simulink model "untitled1"  (Simulink 7.5)
settings: Solver=ode45  StartTime=0.0  StopTime=10.0  RelTol=1e-3
libraries: simulink x4
settings Model: Creator=dell  LastModifiedBy=dell

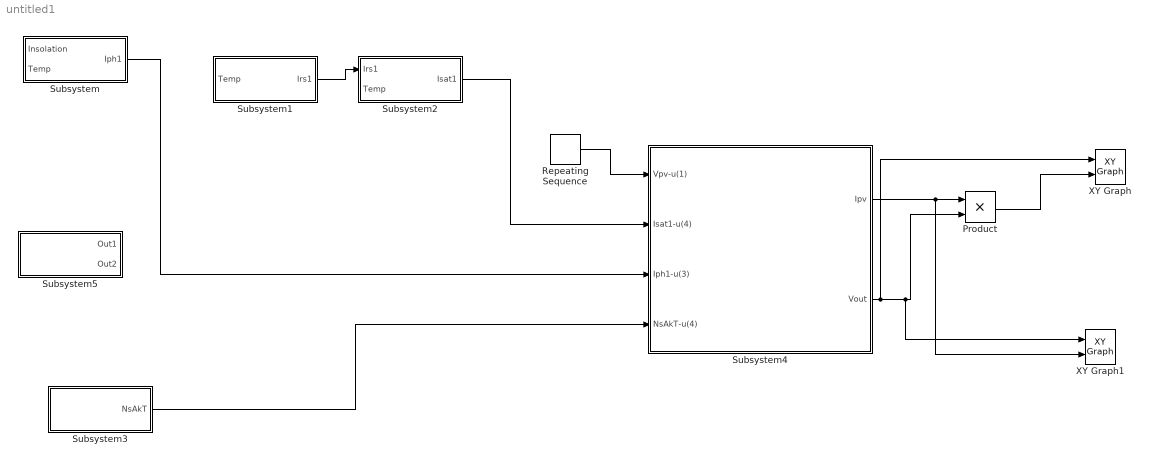
== system untitled1 ==
  Product : Product  OutDataType=fixdt(1, 16)  OutScaling=2^0  RndMeth=Zero
  Repeating Sequence : simulink/Sources/Repeating Sequence  SystemSampleTime=-1  rep_seq_t=[0 12]  rep_seq_y=[0 21.74]
  Subsystem : Subsystem
  Subsystem1 : Subsystem
  Subsystem2 : Subsystem
  Subsystem3 : Subsystem
  Subsystem4 : Subsystem
  Subsystem5 : Subsystem
  XY Graph : simulink/Sinks/XY Graph  SystemSampleTime=-1  xmin=0  xmax=25  ymin=0  ymax=40  st=-1
  XY Graph1 : simulink/Sinks/XY Graph  SystemSampleTime=-1  xmin=0  xmax=25  ymin=0  ymax=5  st=-1
  wires:
  Subsystem/1(Iph1) -> Subsystem4/3(Iph1-u(3))
  Subsystem1/1(Irs1) -> Subsystem2/1(Irs1)
  Subsystem3/1(NsAkT) -> Subsystem4/4(NsAkT-u(4))
  Subsystem2/1(Isat1) -> Subsystem4/2(Isat1-u(4))
  Repeating Sequence/1 -> Subsystem4/1(Vpv-u(1))
  Subsystem4/1(Ipv) -> Product/1, XY Graph1/2
  Subsystem4/2(Vout) -> Product/2, XY Graph1/1, XY Graph/1
  Product/1 -> XY Graph/2

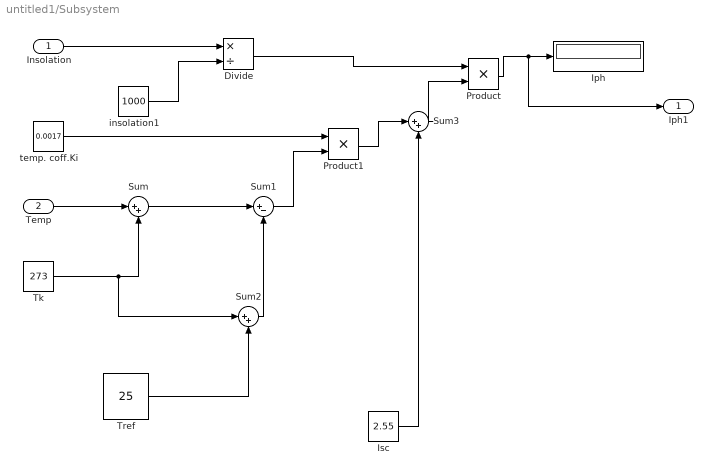
== system untitled1/Subsystem ==
  Insolation : Inport  OutDataType=fixdt(1, 16)  OutScaling=2^0
  Temp : Inport  Port=2  OutDataType=fixdt(1, 16)  OutScaling=2^0
  Divide : Product  Inputs=*/  OutDataType=fixdt(1, 16)  OutScaling=2^-10
  Iph : Display
  Isc : Constant  Value=2.55  OutDataType=fixdt(1, 16)  OutScaling=2^0
  Product : Product  OutDataType=fixdt(1, 16)  OutScaling=2^0  RndMeth=Zero
  Product1 : Product  OutDataType=fixdt(1, 16)  OutScaling=2^0  RndMeth=Zero
  Sum : Sum  Inputs=|++  OutDataType=fixdt(1, 16)  OutScaling=2^0
  Sum1 : Sum  Inputs=|+-  OutDataType=fixdt(1, 16)  OutScaling=2^0
  Sum2 : Sum  Inputs=|++  OutDataType=fixdt(1, 16)  OutScaling=2^0
  Sum3 : Sum  Inputs=|++  OutDataType=fixdt(1, 16)  OutScaling=2^0
  Tk : Constant  Value=273  OutDataType=fixdt(1, 16)  OutScaling=2^0
  Tref : Constant  Value=25  OutDataType=fixdt(1, 16)  OutScaling=2^0
  insolation1 : Constant  Value=1000  OutDataType=fixdt(1, 16)  OutScaling=2^0
  temp. coff.Ki : Constant  Value=0.0017  OutDataType=fixdt(1, 16)  OutScaling=2^0
  Iph1 : Outport  OutDataType=fixdt(1, 16)  OutScaling=2^0
  wires:
  Product/1 -> Iph/1, Iph1/1
  temp. coff.Ki/1 -> Product1/1
  Temp/1 -> Sum/1
  Tk/1 -> Sum/2, Sum2/1
  Sum/1 -> Sum1/1
  Tref/1 -> Sum2/2
  Sum2/1 -> Sum1/2
  Sum1/1 -> Product1/2
  Product1/1 -> Sum3/1
  Isc/1 -> Sum3/2
  Sum3/1 -> Product/2
  Insolation/1 -> Divide/1
  Divide/1 -> Product/1
  insolation1/1 -> Divide/2

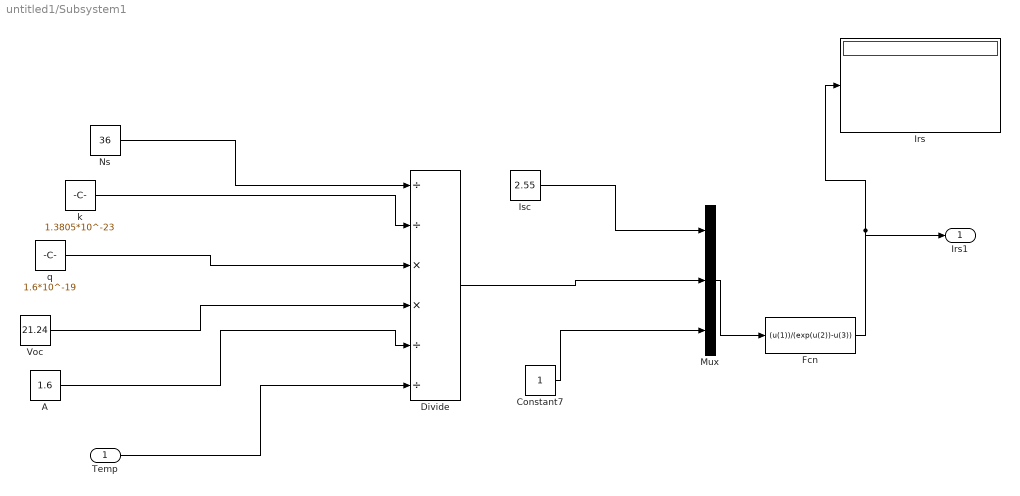
== system untitled1/Subsystem1 ==
  Temp : Inport  OutDataType=fixdt(1, 16)  OutScaling=2^0
  A : Constant  Value=1.6  OutDataType=fixdt(1, 16)  OutScaling=2^0
  Constant7 : Constant  OutDataType=fixdt(1, 16)  OutScaling=2^0
  Divide : Product  Inputs=//**//  OutDataType=fixdt(1, 16)  OutScaling=2^-10
  Fcn : Fcn  Expr=(u(1))/(exp(u(2))-u(3))
  Irs : Display
      settings: Format=short_e
  Isc : Constant  Value=2.55  OutDataType=fixdt(1, 16)  OutScaling=2^0
  Mux : Mux  Inputs=3
  Ns : Constant  Value=36  OutDataType=fixdt(1, 16)  OutScaling=2^0
  Voc : Constant  Value=21.24  OutDataType=fixdt(1, 16)  OutScaling=2^0
  k : Constant  Value=1.3805*10^-23  OutDataType=fixdt(1, 16)  OutScaling=2^0
  q : Constant  Value=1.6*10^-19  OutDataType=fixdt(1, 16)  OutScaling=2^0
  Irs1 : Outport  OutDataType=fixdt(1, 16)  OutScaling=2^0
  wires:
  Ns/1 -> Divide/1
  k/1 -> Divide/2
  q/1 -> Divide/3
  Voc/1 -> Divide/4
  A/1 -> Divide/5
  Temp/1 -> Divide/6
  Isc/1 -> Mux/1
  Divide/1 -> Mux/2
  Mux/1 -> Fcn/1
  Fcn/1 -> Irs/1, Irs1/1
  Constant7/1 -> Mux/3

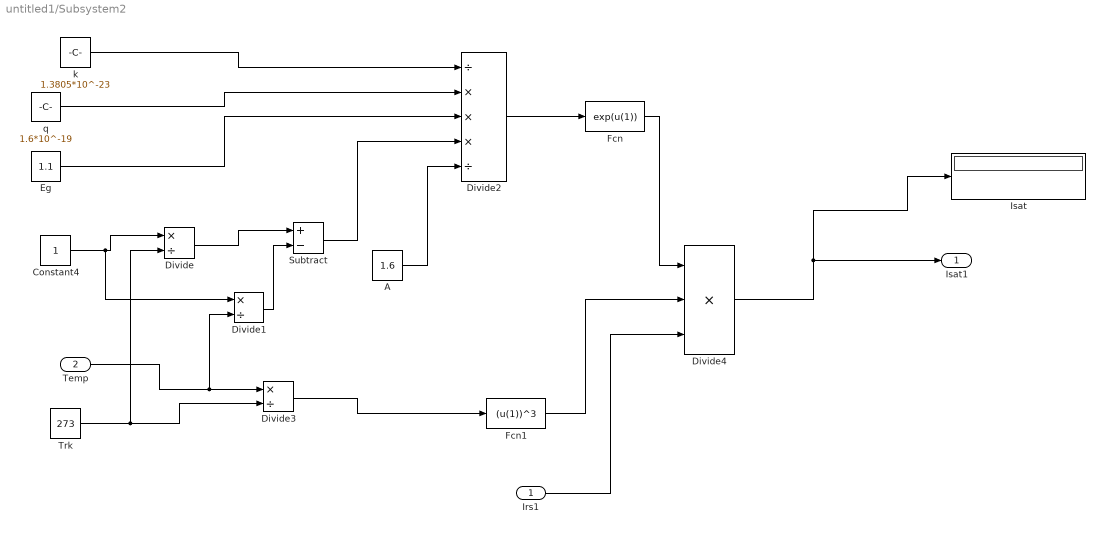
== system untitled1/Subsystem2 ==
  Irs1 : Inport  OutDataType=fixdt(1, 16)  OutScaling=2^0
  Temp : Inport  Port=2  OutDataType=fixdt(1, 16)  OutScaling=2^0
  A : Constant  Value=1.6  OutDataType=fixdt(1, 16)  OutScaling=2^0
  Constant4 : Constant  OutDataType=fixdt(1, 16)  OutScaling=2^0
  Divide : Product  Inputs=*/  OutDataType=fixdt(1, 16)  OutScaling=2^-10
  Divide1 : Product  Inputs=*/  OutDataType=fixdt(1, 16)  OutScaling=2^-10
  Divide2 : Product  Inputs=/***/  OutDataType=fixdt(1, 16)  OutScaling=2^-10
  Divide3 : Product  Inputs=*/  OutDataType=fixdt(1, 16)  OutScaling=2^-10
  Divide4 : Product  Inputs=***  OutDataType=fixdt(1, 16)  OutScaling=2^-10
  Eg : Constant  Value=1.1  OutDataType=fixdt(1, 16)  OutScaling=2^0
  Fcn : Fcn  Expr=exp(u(1))
  Fcn1 : Fcn  Expr=(u(1))^3
  Isat : Display
  Subtract : Sum  Inputs=+-  OutDataType=fixdt(1, 16)  OutScaling=2^-10
  Trk : Constant  Value=273  OutDataType=fixdt(1, 16)  OutScaling=2^0
  k : Constant  Value=1.3805*10^-23  OutDataType=fixdt(1, 16)  OutScaling=2^0
  q : Constant  Value=1.6*10^-19  OutDataType=fixdt(1, 16)  OutScaling=2^0
  Isat1 : Outport  OutDataType=fixdt(1, 16)  OutScaling=2^0
  wires:
  k/1 -> Divide2/1
  q/1 -> Divide2/2
  Eg/1 -> Divide2/3
  Constant4/1 -> Divide/1, Divide1/1
  Temp/1 -> Divide3/1, Divide1/2
  Trk/1 -> Divide3/2, Divide/2
  Divide/1 -> Subtract/1
  Divide1/1 -> Subtract/2
  Subtract/1 -> Divide2/4
  A/1 -> Divide2/5
  Divide2/1 -> Fcn/1
  Divide4/1 -> Isat/1, Isat1/1
  Fcn/1 -> Divide4/1
  Divide3/1 -> Fcn1/1
  Fcn1/1 -> Divide4/2
  Irs1/1 -> Divide4/3

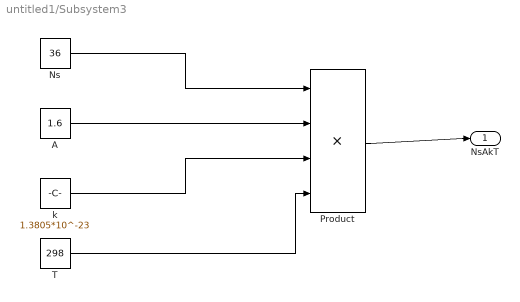
== system untitled1/Subsystem3 ==
  A : Constant  Value=1.6  OutDataType=fixdt(1, 16)  OutScaling=2^0
  Ns : Constant  Value=36  OutDataType=fixdt(1, 16)  OutScaling=2^0
  Product : Product  Inputs=4  OutDataType=fixdt(1, 16)  OutScaling=2^0  RndMeth=Zero
  T : Constant  Value=298  OutDataType=fixdt(1, 16)  OutScaling=2^0
  k : Constant  Value=1.3805*10^-23  OutDataType=fixdt(1, 16)  OutScaling=2^0
  NsAkT : Outport  OutDataType=fixdt(1, 16)  OutScaling=2^0
  wires:
  Ns/1 -> Product/1
  A/1 -> Product/2
  k/1 -> Product/3
  T/1 -> Product/4
  Product/1 -> NsAkT/1

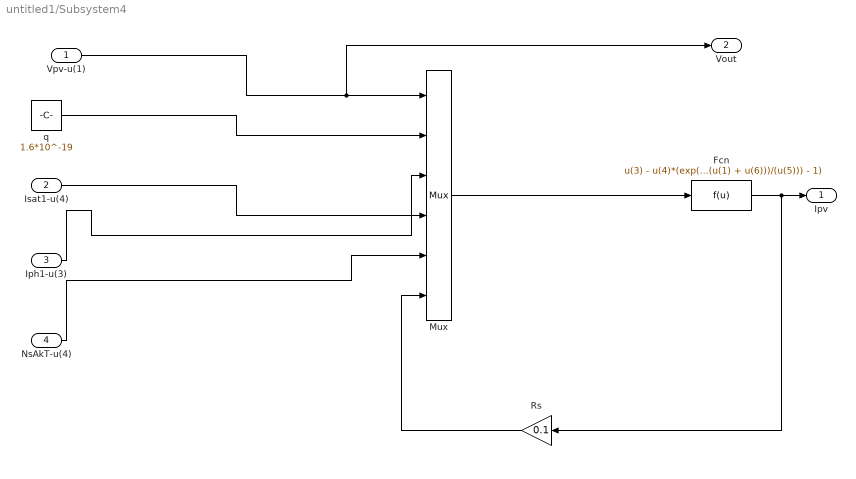
== system untitled1/Subsystem4 ==
  Vpv-u(1) : Inport  OutDataType=fixdt(1, 16)  OutScaling=2^0
  Isat1-u(4) : Inport  Port=2  OutDataType=fixdt(1, 16)  OutScaling=2^0
  Iph1-u(3) : Inport  Port=3  OutDataType=fixdt(1, 16)  OutScaling=2^0
  NsAkT-u(4) : Inport  Port=4  OutDataType=fixdt(1, 16)  OutScaling=2^0
  Fcn : Fcn  Expr=u(3) - u(4)*(exp((u(2)*(u(1) + u(6)))/(u(5))) - 1)
  Mux : Mux  Inputs=6
  Rs : Gain  Gain=0.1  ParameterDataType=fixdt(1, 16)  ParameterScaling=2^0  OutDataType=fixdt(1, 16)  OutScaling=2^0
  q : Constant  Value=1.6*10^-19  OutDataType=fixdt(1, 16)  OutScaling=2^0
  Ipv : Outport  OutDataType=fixdt(1, 16)  OutScaling=2^0
  Vout : Outport  Port=2  OutDataType=fixdt(1, 16)  OutScaling=2^0
  wires:
  Vpv-u(1)/1 -> Mux/1, Vout/1
  q/1 -> Mux/2
  NsAkT-u(4)/1 -> Mux/5
  Mux/1 -> Fcn/1
  Fcn/1 -> Ipv/1, Rs/1
  Isat1-u(4)/1 -> Mux/4
  Iph1-u(3)/1 -> Mux/3
  Rs/1 -> Mux/6

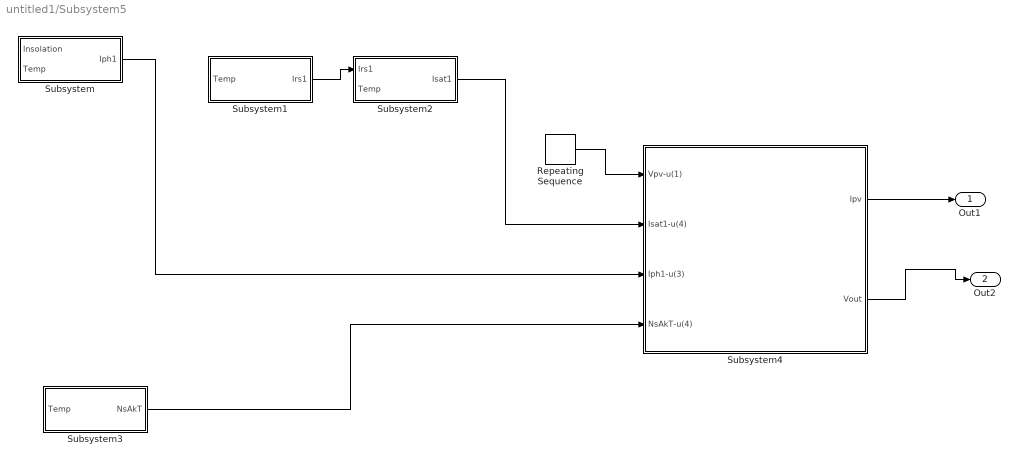
== system untitled1/Subsystem5 ==
  Repeating Sequence : simulink/Sources/Repeating Sequence  SystemSampleTime=-1  rep_seq_t=[0 12]  rep_seq_y=[0 21.74]
  Subsystem : Subsystem
  Subsystem1 : Subsystem
  Subsystem2 : Subsystem
  Subsystem3 : Subsystem
  Subsystem4 : Subsystem
  Out1 : Outport  OutDataType=fixdt(1, 16)  OutScaling=2^0
  Out2 : Outport  Port=2  OutDataType=fixdt(1, 16)  OutScaling=2^0
  wires:
  Subsystem/1(Iph1) -> Subsystem4/3(Iph1-u(3))
  Subsystem1/1(Irs1) -> Subsystem2/1(Irs1)
  Subsystem3/1(NsAkT) -> Subsystem4/4(NsAkT-u(4))
  Subsystem2/1(Isat1) -> Subsystem4/2(Isat1-u(4))
  Repeating Sequence/1 -> Subsystem4/1(Vpv-u(1))
  Subsystem4/1(Ipv) -> Out1/1
  Subsystem4/2(Vout) -> Out2/1

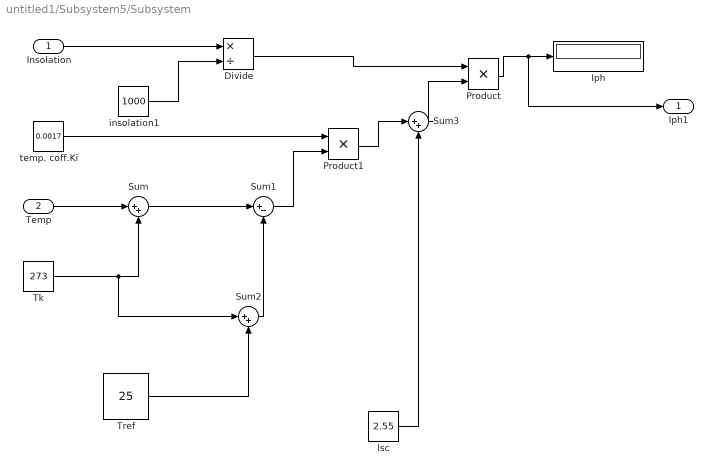
== system untitled1/Subsystem5/Subsystem ==
  Insolation : Inport  OutDataType=fixdt(1, 16)  OutScaling=2^0
  Temp : Inport  Port=2  OutDataType=fixdt(1, 16)  OutScaling=2^0
  Divide : Product  Inputs=*/  OutDataType=fixdt(1, 16)  OutScaling=2^-10
  Iph : Display
  Isc : Constant  Value=2.55  OutDataType=fixdt(1, 16)  OutScaling=2^0
  Product : Product  OutDataType=fixdt(1, 16)  OutScaling=2^0  RndMeth=Zero
  Product1 : Product  OutDataType=fixdt(1, 16)  OutScaling=2^0  RndMeth=Zero
  Sum : Sum  Inputs=|++  OutDataType=fixdt(1, 16)  OutScaling=2^0
  Sum1 : Sum  Inputs=|+-  OutDataType=fixdt(1, 16)  OutScaling=2^0
  Sum2 : Sum  Inputs=|++  OutDataType=fixdt(1, 16)  OutScaling=2^0
  Sum3 : Sum  Inputs=|++  OutDataType=fixdt(1, 16)  OutScaling=2^0
  Tk : Constant  Value=273  OutDataType=fixdt(1, 16)  OutScaling=2^0
  Tref : Constant  Value=25  OutDataType=fixdt(1, 16)  OutScaling=2^0
  insolation1 : Constant  Value=1000  OutDataType=fixdt(1, 16)  OutScaling=2^0
  temp. coff.Ki : Constant  Value=0.0017  OutDataType=fixdt(1, 16)  OutScaling=2^0
  Iph1 : Outport  OutDataType=fixdt(1, 16)  OutScaling=2^0
  wires:
  Product/1 -> Iph/1, Iph1/1
  temp. coff.Ki/1 -> Product1/1
  Temp/1 -> Sum/1
  Tk/1 -> Sum/2, Sum2/1
  Sum/1 -> Sum1/1
  Tref/1 -> Sum2/2
  Sum2/1 -> Sum1/2
  Sum1/1 -> Product1/2
  Product1/1 -> Sum3/1
  Isc/1 -> Sum3/2
  Sum3/1 -> Product/2
  Insolation/1 -> Divide/1
  Divide/1 -> Product/1
  insolation1/1 -> Divide/2

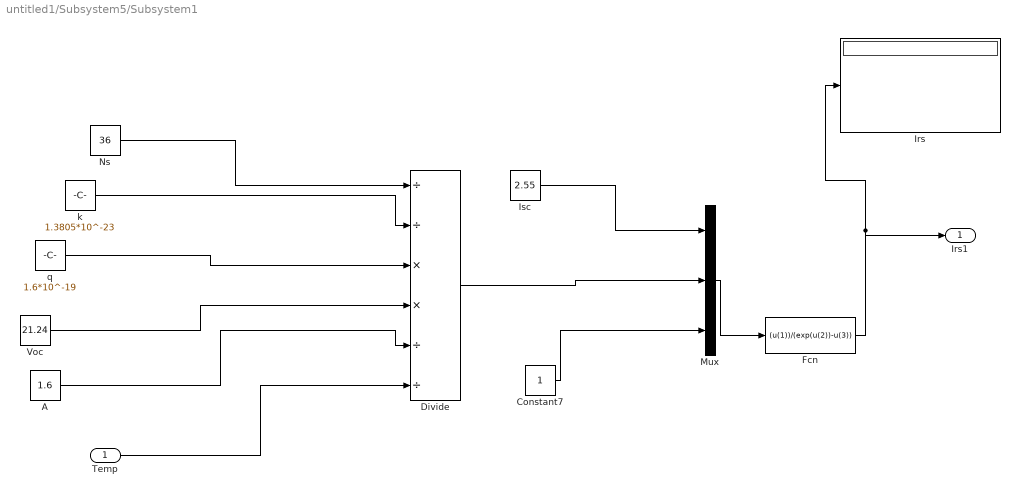
== system untitled1/Subsystem5/Subsystem1 ==
  Temp : Inport  OutDataType=fixdt(1, 16)  OutScaling=2^0
  A : Constant  Value=1.6  OutDataType=fixdt(1, 16)  OutScaling=2^0
  Constant7 : Constant  OutDataType=fixdt(1, 16)  OutScaling=2^0
  Divide : Product  Inputs=//**//  OutDataType=fixdt(1, 16)  OutScaling=2^-10
  Fcn : Fcn  Expr=(u(1))/(exp(u(2))-u(3))
  Irs : Display
      settings: Format=short_e
  Isc : Constant  Value=2.55  OutDataType=fixdt(1, 16)  OutScaling=2^0
  Mux : Mux  Inputs=3
  Ns : Constant  Value=36  OutDataType=fixdt(1, 16)  OutScaling=2^0
  Voc : Constant  Value=21.24  OutDataType=fixdt(1, 16)  OutScaling=2^0
  k : Constant  Value=1.3805*10^-23  OutDataType=fixdt(1, 16)  OutScaling=2^0
  q : Constant  Value=1.6*10^-19  OutDataType=fixdt(1, 16)  OutScaling=2^0
  Irs1 : Outport  OutDataType=fixdt(1, 16)  OutScaling=2^0
  wires:
  Ns/1 -> Divide/1
  k/1 -> Divide/2
  q/1 -> Divide/3
  Voc/1 -> Divide/4
  A/1 -> Divide/5
  Temp/1 -> Divide/6
  Isc/1 -> Mux/1
  Divide/1 -> Mux/2
  Mux/1 -> Fcn/1
  Fcn/1 -> Irs/1, Irs1/1
  Constant7/1 -> Mux/3

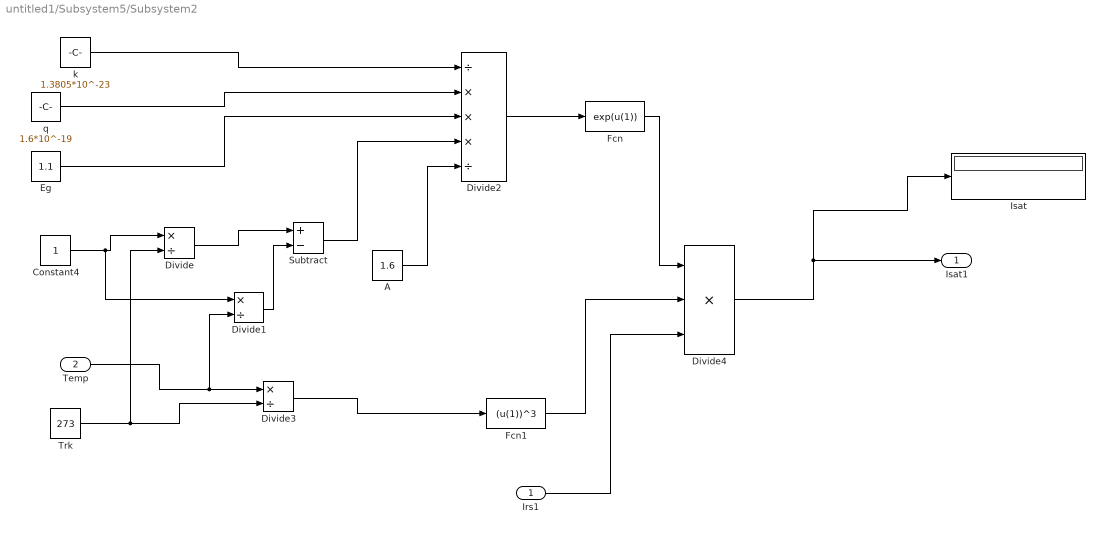
== system untitled1/Subsystem5/Subsystem2 ==
  Irs1 : Inport  OutDataType=fixdt(1, 16)  OutScaling=2^0
  Temp : Inport  Port=2  OutDataType=fixdt(1, 16)  OutScaling=2^0
  A : Constant  Value=1.6  OutDataType=fixdt(1, 16)  OutScaling=2^0
  Constant4 : Constant  OutDataType=fixdt(1, 16)  OutScaling=2^0
  Divide : Product  Inputs=*/  OutDataType=fixdt(1, 16)  OutScaling=2^-10
  Divide1 : Product  Inputs=*/  OutDataType=fixdt(1, 16)  OutScaling=2^-10
  Divide2 : Product  Inputs=/***/  OutDataType=fixdt(1, 16)  OutScaling=2^-10
  Divide3 : Product  Inputs=*/  OutDataType=fixdt(1, 16)  OutScaling=2^-10
  Divide4 : Product  Inputs=***  OutDataType=fixdt(1, 16)  OutScaling=2^-10
  Eg : Constant  Value=1.1  OutDataType=fixdt(1, 16)  OutScaling=2^0
  Fcn : Fcn  Expr=exp(u(1))
  Fcn1 : Fcn  Expr=(u(1))^3
  Isat : Display
  Subtract : Sum  Inputs=+-  OutDataType=fixdt(1, 16)  OutScaling=2^-10
  Trk : Constant  Value=273  OutDataType=fixdt(1, 16)  OutScaling=2^0
  k : Constant  Value=1.3805*10^-23  OutDataType=fixdt(1, 16)  OutScaling=2^0
  q : Constant  Value=1.6*10^-19  OutDataType=fixdt(1, 16)  OutScaling=2^0
  Isat1 : Outport  OutDataType=fixdt(1, 16)  OutScaling=2^0
  wires:
  k/1 -> Divide2/1
  q/1 -> Divide2/2
  Eg/1 -> Divide2/3
  Constant4/1 -> Divide/1, Divide1/1
  Temp/1 -> Divide3/1, Divide1/2
  Trk/1 -> Divide3/2, Divide/2
  Divide/1 -> Subtract/1
  Divide1/1 -> Subtract/2
  Subtract/1 -> Divide2/4
  A/1 -> Divide2/5
  Divide2/1 -> Fcn/1
  Divide4/1 -> Isat/1, Isat1/1
  Fcn/1 -> Divide4/1
  Divide3/1 -> Fcn1/1
  Fcn1/1 -> Divide4/2
  Irs1/1 -> Divide4/3

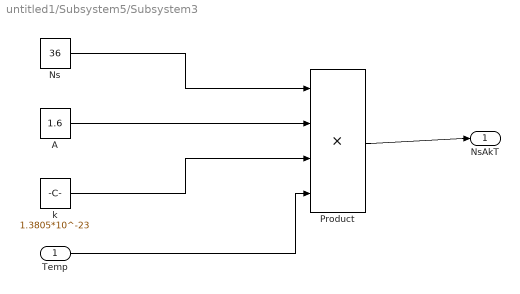
== system untitled1/Subsystem5/Subsystem3 ==
  Temp : Inport  OutDataType=fixdt(1, 16)  OutScaling=2^0
  A : Constant  Value=1.6  OutDataType=fixdt(1, 16)  OutScaling=2^0
  Ns : Constant  Value=36  OutDataType=fixdt(1, 16)  OutScaling=2^0
  Product : Product  Inputs=4  OutDataType=fixdt(1, 16)  OutScaling=2^0  RndMeth=Zero
  k : Constant  Value=1.3805*10^-23  OutDataType=fixdt(1, 16)  OutScaling=2^0
  NsAkT : Outport  OutDataType=fixdt(1, 16)  OutScaling=2^0
  wires:
  Ns/1 -> Product/1
  A/1 -> Product/2
  k/1 -> Product/3
  Temp/1 -> Product/4
  Product/1 -> NsAkT/1

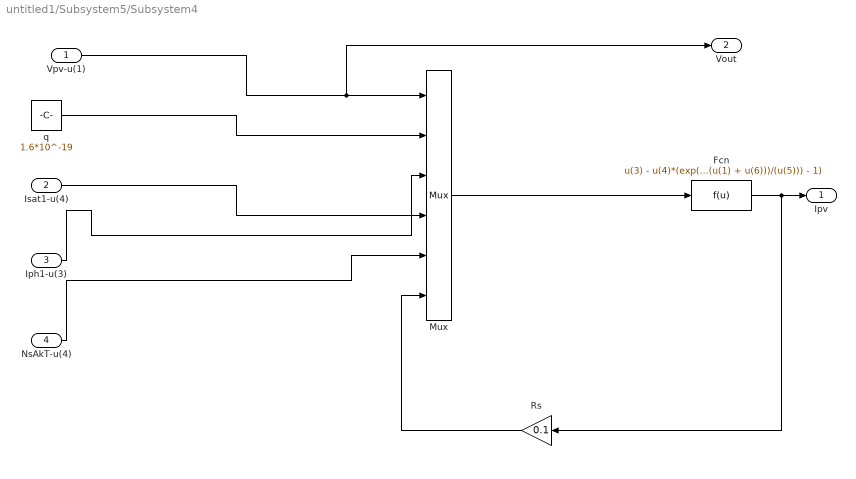
== system untitled1/Subsystem5/Subsystem4 ==
  Vpv-u(1) : Inport  OutDataType=fixdt(1, 16)  OutScaling=2^0
  Isat1-u(4) : Inport  Port=2  OutDataType=fixdt(1, 16)  OutScaling=2^0
  Iph1-u(3) : Inport  Port=3  OutDataType=fixdt(1, 16)  OutScaling=2^0
  NsAkT-u(4) : Inport  Port=4  OutDataType=fixdt(1, 16)  OutScaling=2^0
  Fcn : Fcn  Expr=u(3) - u(4)*(exp((u(2)*(u(1) + u(6)))/(u(5))) - 1)
  Mux : Mux  Inputs=6
  Rs : Gain  Gain=0.1  ParameterDataType=fixdt(1, 16)  ParameterScaling=2^0  OutDataType=fixdt(1, 16)  OutScaling=2^0
  q : Constant  Value=1.6*10^-19  OutDataType=fixdt(1, 16)  OutScaling=2^0
  Ipv : Outport  OutDataType=fixdt(1, 16)  OutScaling=2^0
  Vout : Outport  Port=2  OutDataType=fixdt(1, 16)  OutScaling=2^0
  wires:
  Vpv-u(1)/1 -> Mux/1, Vout/1
  q/1 -> Mux/2
  NsAkT-u(4)/1 -> Mux/5
  Mux/1 -> Fcn/1
  Fcn/1 -> Ipv/1, Rs/1
  Isat1-u(4)/1 -> Mux/4
  Iph1-u(3)/1 -> Mux/3
  Rs/1 -> Mux/6
